simulink model "prob3"  (R2020b)
settings: Solver=VariableStepAuto  StartTime=0.0  StopTime=1  FixedStep=0.001  RelTol=1e-3
model workspace: external: MATLAB File C:\Users\deves\MATLAB\Projects\problem3\data3.m (data not in the file)
settings Model: Creator=deves  LastModifiedBy=deves
settings DataIOCC: ExternalInput=[t, f]  SaveFormat=Array  SignalLogging=off  DSMLogging=off  ReturnWorkspaceOutputs=off

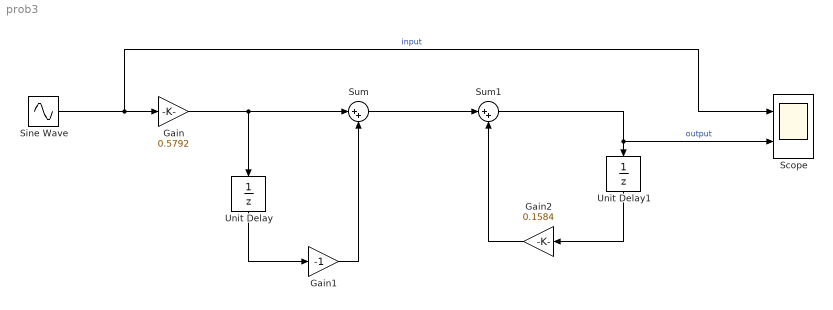
== system prob3 ==
  Gain : Gain  Gain=0.5792
  Gain1 : Gain  Gain=-1
  Gain2 : Gain  Gain=0.1584
  Scope : Scope  NumInputPorts=2
  Sine Wave : Sin  Amplitude=2  Frequency=10000*2*pi  SampleTime=0
  Sum : Sum  Inputs=|++
  Sum1 : Sum  Inputs=|++
  Unit Delay : UnitDelay  SampleTime=-1  HasFrameUpgradeWarning=on
  Unit Delay1 : UnitDelay  SampleTime=-1  HasFrameUpgradeWarning=on
  wires:
  Gain/1 -> Unit Delay/1, Sum/1
  Sum/1 -> Sum1/1
  Sum1/1 -> Unit Delay1/1, Scope/2  "output"
  Unit Delay1/1 -> Gain2/1
  Gain2/1 -> Sum1/2
  Gain1/1 -> Sum/2
  Unit Delay/1 -> Gain1/1
  Sine Wave/1 -> Scope/1, Gain/1  "input"
